simulink model "Genset"  (R2019b)
settings: Solver=VariableStepAuto  StartTime=0.0  StopTime=tEnd  RelTol=1e-3
values from neighbouring files (symbols this model uses):
  etaGenGR = 0.93    [main.m]
  genMotorData = load(GENERATOR_MOTOR_DATA_NAME)    [main.m]
  GRgen = 1.4    [main.m]
  initialGasVolume = 5    [main.m]
  k_gal2kWh = 32.3    [main.m]
  k_hr2s = 3600    [main.m]
  k_m32gal = 264.172    [main.m]
  k_rpm2rps = 2*pi()/60    [main.m]
  k_W2kW = 1/1000    (= 0.001)    [main.m]
libraries: autolibsharedmappedengines x1
(part 1 of 3)
settings Model: Creator=Chris  LastModifiedBy=Chris

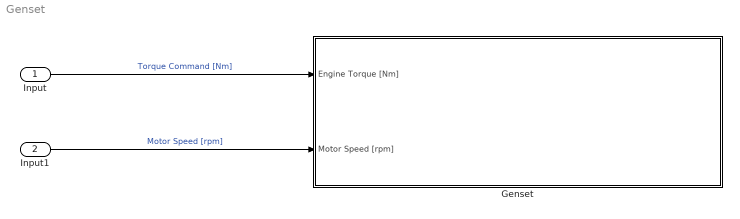
== system Genset ==
  Input : Inport
  Input1 : Inport  Port=2
  Genset : Subsystem
  wires:
  Input/1 -> Genset/1(Engine Torque [Nm])  "Torque Command [Nm]"
  Input1/1 -> Genset/2(Motor Speed [rpm])  "Motor Speed [rpm]"

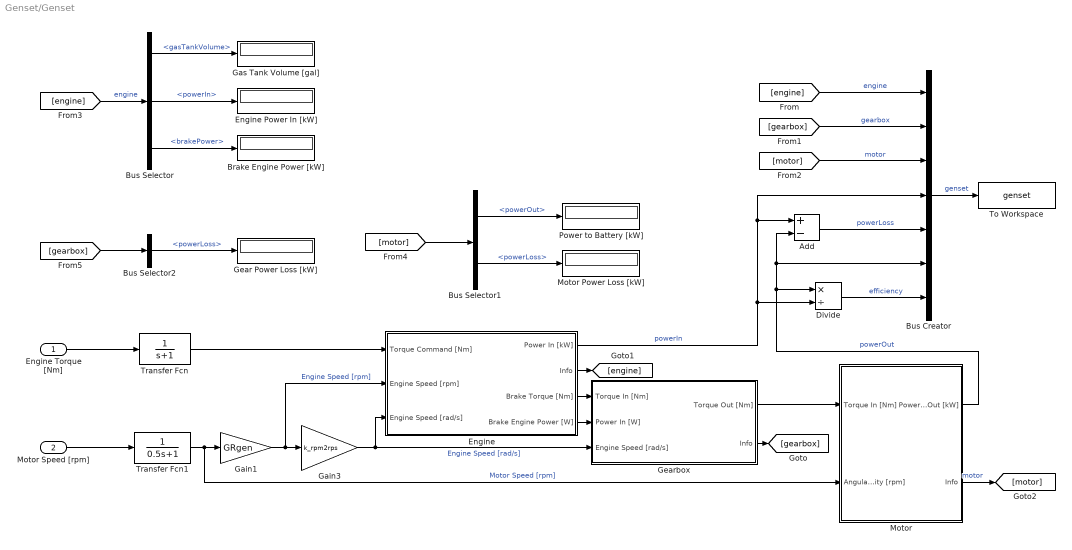
== system Genset/Genset ==
  Engine Torque [Nm] : Inport
  Motor Speed [rpm] : Inport  Port=2
  Add : Sum  Inputs=+-
  Brake Engine Power [kW] : Display
  Bus Creator : BusCreator  Inputs=7
  Bus Selector : BusSelector  OutputSignals=gasTankVolume,powerIn,brakePower
  Bus Selector1 : BusSelector  OutputSignals=powerOut,powerLoss
  Bus Selector2 : BusSelector  OutputSignals=powerLoss
  Divide : Product  Inputs=*/
  Engine : Subsystem
  Engine Power In [kW] : Display
  Gain1 : Gain  Gain=GRgen
  Gain3 : Gain  Gain=k_rpm2rps
  Gas Tank Volume [gal] : Display
  Gear Power Loss [kW] : Display
  Gearbox : Subsystem
  Motor : Subsystem
  Motor Power Loss [kW] : Display
  Power to Battery [kW] : Display
  To Workspace : ToWorkspace  VariableName=genset  SaveFormat=Timeseries  SampleTime=-1
  Transfer Fcn : TransferFcn  Denominator=[1 1]
  Transfer Fcn1 : TransferFcn  Denominator=[0.5 1]
  wires:
  Bus Selector/1 -> Gas Tank Volume [gal]/1  "<gasTankVolume>"
  Motor Speed [rpm]/1 -> Transfer Fcn1/1
  Motor/2(Info) -> [motor]  "motor"
  [motor] -> Bus Selector1/1
  Bus Selector1/2 -> Motor Power Loss [kW]/1  "<powerLoss>"
  [engine] -> Bus Selector/1  "engine"
  Bus Selector2/1 -> Gear Power Loss [kW]/1  "<powerLoss>"
  Engine Torque [Nm]/1 -> Transfer Fcn/1
  Bus Selector/3 -> Brake Engine Power [kW]/1  "<brakePower>"
  Bus Selector1/1 -> Power to Battery [kW]/1  "<powerOut>"
  Engine/1(Power In [kW]) -> Divide/2, Bus Creator/4, Add/1  "powerIn"
  [gearbox] -> Bus Selector2/1
  Bus Selector/2 -> Engine Power In [kW]/1  "<powerIn>"
  Divide/1 -> Bus Creator/7  "efficiency"
  Gain1/1 -> Engine/2(Engine Speed [rpm]), Gain3/1  "Engine Speed [rpm]"
  Transfer Fcn1/1 -> Motor/2(Angular Velocity [rpm]), Gain1/1  "Motor Speed [rpm]"
  Add/1 -> Bus Creator/5  "powerLoss"
  Engine/3(Brake Torque [Nm]) -> Gearbox/1(Torque In [Nm])
  Gain3/1 -> Engine/3(Engine Speed [rad/s]), Gearbox/3(Engine Speed [rad/s])  "Engine Speed [rad/s]"
  Gearbox/1(Torque Out [Nm]) -> Motor/1(Torque In [Nm])
  [motor] -> Bus Creator/3  "motor"
  [gearbox] -> Bus Creator/2  "gearbox"
  Motor/1(Power Out [kW]) -> Bus Creator/6, Add/2, Divide/1  "powerOut"
  Gearbox/2(Info) -> [gearbox]
  [engine] -> Bus Creator/1  "engine"
  Engine/2(Info) -> [engine]
  Bus Creator/1 -> To Workspace/1  "genset"
  Engine/4(Brake Engine Power [W]) -> Gearbox/2(Power In [W])
  Transfer Fcn/1 -> Engine/1(Torque Command [Nm])
